simulink model "Simulink_pid_program"  (R2017b)
settings: Solver=FixedStepDiscrete  StartTime=0.0  StopTime=Inf  RelTol=1e-3  EnableMultiTasking=on
undefined symbols (not defined in the file or in its folder): serial
libraries: instrumentlib x3
settings Model: Creator=yecheng  LastModifiedBy=Alexander
settings DataIOCC: LimitDataPoints=on  SaveFormat=Array
settings OptimizationCC: LifeSpan=inf
settings DebuggingCC: SolverPrmCheckMsg=warning  SFUnexpectedBacktrackingDiag=warning  SFNoUnconditionalDefaultTransitionDiag=warning  SFExecutionAtInitializationDiag=none
settings HardwareCC: ProdBitPerPointer=32  ProdBitPerSizeT=32  ProdBitPerPtrDiffT=32  ProdLargestAtomicFloat=None  ProdIntDivRoundTo=Undefined  ProdEndianess=Unspecified  ProdWordSize=32  ProdHWDeviceType=32-bit Generic
settings ModelReferenceCC: PropagateSignalLabelsOutOfModel=off
settings CodeAppCC: StateflowObjectComments=on
settings GRTTargetCC: TargetLangStandard=C89/C90 (ANSI)  GeneratePreprocessorConditionals=Disable all
settings ConfigComp: CovMetricSettings=dw  CovHtmlReporting=on  CovSaveCumulativeToWorkspaceVar=on  CovSaveSingleToWorkspaceVar=on  CovExternalEMLEnable=off  CovSFcnEnable=off

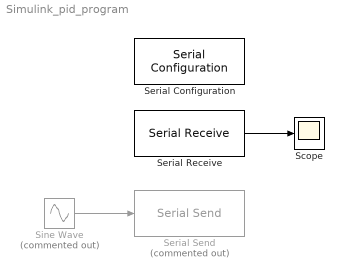
== system Simulink_pid_program ==
  Scope : Scope
  Serial Configuration : instrumentlib/Serial Configuration  Priority=-200000  ComPortMenu=COM5  ComPort=COM4  ObjConstructor=serial('COM4');  BaudRate=9600  DataBits=8  Parity=none  FlowControl=hardware  Timeout=10  ByteOrder=LittleEndian
  Serial Receive : instrumentlib/Serial Receive  ComPortMenu=<Please select a port...>  ComPort=COM4  ObjConstructor=serial('COM4');  Terminator=<none>  DataSize=1  DataType=int32  EnableBlockingMode=on  ActionDataUnavailable=Error  CustomValue=300  SampleTime=0.05
  Serial Send : instrumentlib/Serial Send  Commented=on  ComPortMenu=<Please select a port...>  ComPort=COM4  ObjConstructor=serial('COM4');  Terminator=<none>  EnableBlockingMode=on
  Sine Wave : Sin  Commented=on  SineType=Sample based  Amplitude=100  SampleTime=0.02
  wires:
  Sine Wave/1 -> Serial Send/1
  Serial Receive/1 -> Scope/1
